simulink model "biquad_test_v6_old_IP"  (R2024b)
settings: Solver=FixedStepDiscrete  StartTime=0.0  StopTime=T  RelTol=1e-12
values from neighbouring files (symbols this model uses):
  Fs = 44100    [Biquad_Test_Filter_v3.m]    (also in Biquad_Test_Filter_v4.m; Biquad_Test_Filter_v4_test.m; Biquad_Test_Filter_v5_test.m; Biquad_Test_Filter_v6_test.m)
  g = G_TP    [FilterDesign_v1.m]    (also in FilterDesign_v2.m = ones(3,1); FilterDesign_v3.m; FilterDesign_v4.m = G_BS)
  sos = [SOS_TP(1,1:3)*G_TP(1,1),SOS_TP(1,4:6),SOS_TP(2,1:3)*G_TP(2,1),SOS_TP(2,4:6)]    [FilterDesign_v1.m]    (also in FilterDesign_v2.m = zeros(2,6); FilterDesign_v3.m = SOS_TP; FilterDesign_v4.m = SOS_BS)
  x = 2*sin(2*pi*500*t)+1*sin(2*pi*5000*t)    [Biquad_Test_Filter_v3.m]    (also in Biquad_Test_Filter_v4.m = sin(2*pi*1000*t)+sin(2*pi*50*t); Biquad_Test_Filter_v4_test.m = sin(2*pi*1000*t)+sin(2*pi*50*t); Biquad_Test_Filter_v5_test.m = sin(2*pi*1000*t)+sin(2*pi*50*t); Biquad_Test_Filter_v6_test.m = sin(2*pi*1000*t)+sin(2*pi*50*t))
libraries: dsphdlfiltering2 x2, dspsrcs4 x2
settings Model: DataTypeOverride=Off  Creator=korvo  LastModifiedBy=korvo
settings OptimizationCC: BlockReduction=off  ConditionallyExecuteInputs=off  DefaultParameterBehavior=Inlined  InheritOutputTypeSmallerThanSingle=on
settings DebuggingCC: AlgebraicLoopMsg=error  ArtificialAlgebraicLoopMsg=error  SingleTaskRateTransMsg=error  UnconnectedInputMsg=warning  UnconnectedOutputMsg=warning  UnconnectedLineMsg=warning
settings HardwareCC: ProdBitPerPointer=32  ProdBitPerSizeT=32  ProdBitPerPtrDiffT=32  ProdLargestAtomicFloat=None  ProdIntDivRoundTo=Undefined  ProdEndianess=Unspecified  ProdWordSize=32  ProdHWDeviceType=ASIC/FPGA->ASIC/FPGA  TargetBitPerPointer=64  TargetBitPerSizeT=64  TargetBitPerPtrDiffT=64  TargetLongLongMode=on  TargetIntDivRoundTo=Zero  TargetEndianess=LittleEndian  TargetWordSize=64  TargetHWDeviceType=Custom Processor->MATLAB Host Computer  ProdEqTarget=off

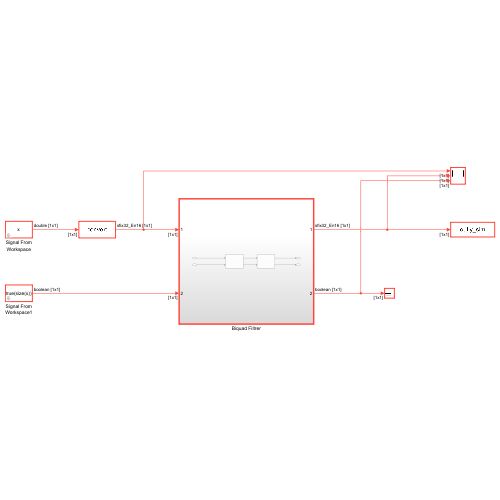
[thumbnail: Simulink's stored preview of the top-level diagram]
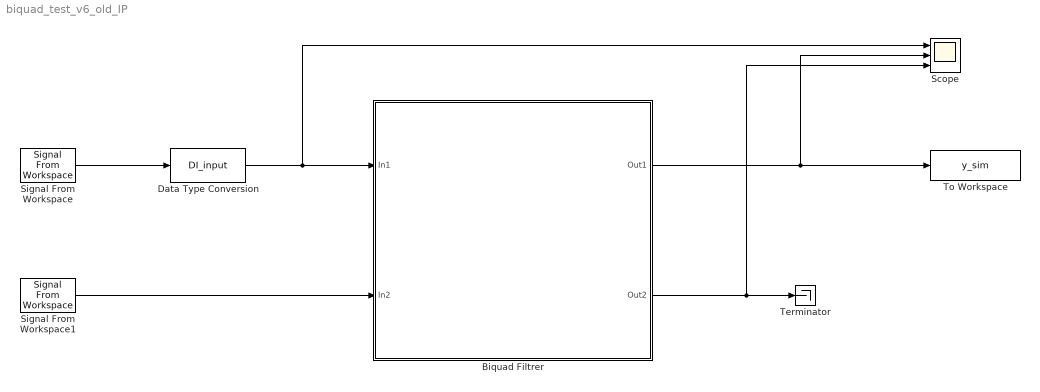
== system biquad_test_v6_old_IP ==
  Biquad Filtrer : Subsystem  TreatAsAtomicUnit=on
  Data Type Conversion : DataTypeConversion  OutDataTypeStr=DI_input  SaturateOnIntegerOverflow=off  RndMeth=Floor
  Scope : Scope  NumInputPorts=3
  Signal From Workspace : dspsrcs4/Signal From Workspace  X=x  Ts=1/Fs  nsamps=1  OutputAfterFinalValue=Setting to zero  ignoreOrWarnInputAndFrameLengths=off  OutputFrames=off
  Signal From Workspace1 : dspsrcs4/Signal From Workspace  X=true(size(x))  Ts=1/Fs  nsamps=1  OutputAfterFinalValue=Setting to zero  ignoreOrWarnInputAndFrameLengths=off  OutputFrames=off
  Terminator : Terminator
  To Workspace : ToWorkspace  VariableName=y_sim  SampleTime=-1
      settings: Save2DSignal=2-D array (concatenate along first dimension)
  wires:
  Signal From Workspace/1 -> Data Type Conversion/1
  Biquad Filtrer/1(Out1) -> Scope/2, To Workspace/1
  Biquad Filtrer/2(Out2) -> Scope/3, Terminator/1
  Data Type Conversion/1 -> Scope/1, Biquad Filtrer/1(In1)
  Signal From Workspace1/1 -> Biquad Filtrer/2(In2)

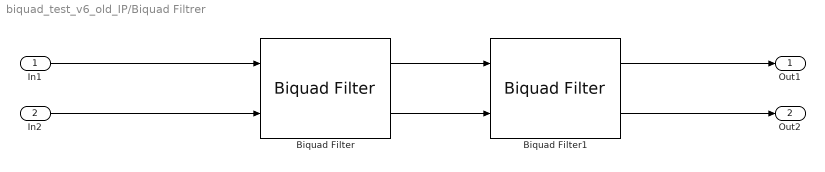
== system biquad_test_v6_old_IP/Biquad Filtrer ==
  In1 : Inport
  In2 : Inport  Port=2
  Biquad Filter : dsphdlfiltering2/Biquad Filter  Structure=Direct form II  Numerator=sos(1,1:3)  Denominator=sos(1,4:6)  ScaleValues=[ g]  SimulateUsing=Code generation  roundingMode=Floor  overflowMode=off  NumeratorDataTypeStr=Inherit: Same word length as input  DenominatorDataTypeStr=Inherit: Same word length as input  ScaleValuesDataTypeStr=Inherit: Same word length as input  CoefficientsDataTypeStr=Inherit: Same word length as input
  Biquad Filter1 : dsphdlfiltering2/Biquad Filter  Structure=Direct form II  Numerator=sos(2,1:3)  Denominator=sos(2,4:6)  ScaleValues=1  SimulateUsing=Code generation  roundingMode=Floor  overflowMode=off  NumeratorDataTypeStr=Inherit: Same word length as input  DenominatorDataTypeStr=Inherit: Same word length as input  ScaleValuesDataTypeStr=Inherit: Same word length as input  CoefficientsDataTypeStr=Inherit: Same word length as input
  Out1 : Outport
  Out2 : Outport  Port=2
  wires:
  In1/1 -> Biquad Filter/1
  Biquad Filter/1 -> Biquad Filter1/1
  In2/1 -> Biquad Filter/2
  Biquad Filter/2 -> Biquad Filter1/2
  Biquad Filter1/1 -> Out1/1
  Biquad Filter1/2 -> Out2/1
